simulink model "FO_CTDNN_P_Bia_Para_0_V1"  (R2021b)
settings: Solver=ode5  StartTime=0.0  StopTime=40  FixedStep=0.005  RelTol=1e-3
(part 1 of 2)
settings Model: Creator=a1752760  LastModifiedBy=a1752760
settings SolverCC: AlgebraicLoopSolver=TrustRegion
settings DebuggingCC: SFMachineParentedDataDiag=warning

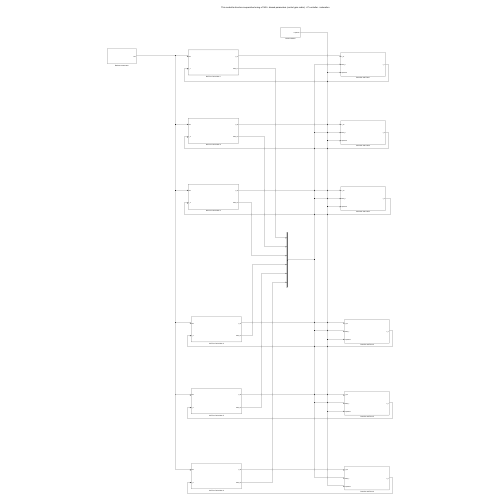
[thumbnail: Simulink's stored preview of the top-level diagram]
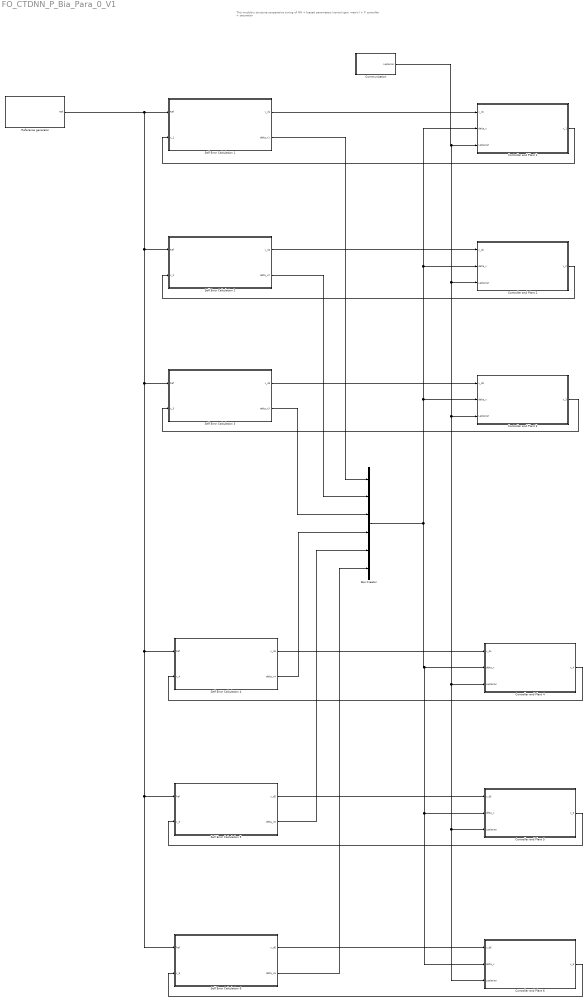
== system FO_CTDNN_P_Bia_Para_0_V1 ==
  note: This module's structure:cooperative tuning of NN + biased parameters (control gain matrix) + P controller + saturation
  Bus Creator : BusCreator  Inputs=6
  Communication : Subsystem
  Controller and Plant 1 : Subsystem  mask{InitialCondition=[-0.2;-0.7;-pi/4], UpperLimit=0.25, LowerLimit=-0.25}
      mask prompts: InitialCondition "Simulink:blkprm_prompts:IntegratorInitCond"; UpperLimit "Simulink:blkprm_prompts:SaturateUpLim"; LowerLimit "Simulink:blkprm_prompts:SaturateLowLim"
      mask TypeOptions InitialCondition: x_int/InitialCondition
      mask TypeOptions UpperLimit: Saturation/UpperLimit
      mask TypeOptions LowerLimit: Saturation/LowerLimit
      mask DialogControl InitialCondition Prompt: Initial condition:
      mask DialogControl UpperLimit Prompt: Upper limit:
      mask DialogControl LowerLimit Prompt: Lower limit:
  Controller and Plant 2 : Subsystem  mask{InitialCondition=[1.6;3.6;-pi/5], UpperLimit=0.25, LowerLimit=-0.25}
      mask prompts: InitialCondition "Simulink:blkprm_prompts:IntegratorInitCond"; UpperLimit "Simulink:blkprm_prompts:SaturateUpLim"; LowerLimit "Simulink:blkprm_prompts:SaturateLowLim"
      mask TypeOptions InitialCondition: x_int/InitialCondition
      mask TypeOptions UpperLimit: Saturation/UpperLimit
      mask TypeOptions LowerLimit: Saturation/LowerLimit
      mask DialogControl InitialCondition Prompt: Initial condition:
      mask DialogControl UpperLimit Prompt: Upper limit:
      mask DialogControl LowerLimit Prompt: Lower limit:
  Controller and Plant 3 : Subsystem  mask{InitialCondition=[-4;-2.4;pi/3], UpperLimit=0.25, LowerLimit=-0.25}
      mask prompts: InitialCondition "Simulink:blkprm_prompts:IntegratorInitCond"; UpperLimit "Simulink:blkprm_prompts:SaturateUpLim"; LowerLimit "Simulink:blkprm_prompts:SaturateLowLim"
      mask TypeOptions InitialCondition: x_int/InitialCondition
      mask TypeOptions UpperLimit: Saturation/UpperLimit
      mask TypeOptions LowerLimit: Saturation/LowerLimit
      mask DialogControl InitialCondition Prompt: Initial condition:
      mask DialogControl UpperLimit Prompt: Upper limit:
      mask DialogControl LowerLimit Prompt: Lower limit:
  Controller and Plant 4 : Subsystem  mask{InitialCondition=[-1.9;-1.1;pi/4], UpperLimit=0.25, LowerLimit=-0.25}
      mask prompts: InitialCondition "Simulink:blkprm_prompts:IntegratorInitCond"; UpperLimit "Simulink:blkprm_prompts:SaturateUpLim"; LowerLimit "Simulink:blkprm_prompts:SaturateLowLim"
      mask TypeOptions InitialCondition: x_int/InitialCondition
      mask TypeOptions UpperLimit: Saturation/UpperLimit
      mask TypeOptions LowerLimit: Saturation/LowerLimit
      mask DialogControl InitialCondition Prompt: Initial condition:
      mask DialogControl UpperLimit Prompt: Upper limit:
      mask DialogControl LowerLimit Prompt: Lower limit:
  Controller and Plant 5 : Subsystem  mask{InitialCondition=[-1.6;-4.6;-pi/3], UpperLimit=0.25, LowerLimit=-0.25}
      mask prompts: InitialCondition "Simulink:blkprm_prompts:IntegratorInitCond"; UpperLimit "Simulink:blkprm_prompts:SaturateUpLim"; LowerLimit "Simulink:blkprm_prompts:SaturateLowLim"
      mask TypeOptions InitialCondition: x_int/InitialCondition
      mask TypeOptions UpperLimit: Saturation/UpperLimit
      mask TypeOptions LowerLimit: Saturation/LowerLimit
      mask DialogControl InitialCondition Prompt: Initial condition:
      mask DialogControl UpperLimit Prompt: Upper limit:
      mask DialogControl LowerLimit Prompt: Lower limit:
  Controller and Plant 6 : Subsystem  mask{InitialCondition=[3.6;-1.5;-pi/6], UpperLimit=0.25, LowerLimit=-0.25}
      mask prompts: InitialCondition "Simulink:blkprm_prompts:IntegratorInitCond"; UpperLimit "Simulink:blkprm_prompts:SaturateUpLim"; LowerLimit "Simulink:blkprm_prompts:SaturateLowLim"
      mask TypeOptions InitialCondition: x_int/InitialCondition
      mask TypeOptions UpperLimit: Saturation/UpperLimit
      mask TypeOptions LowerLimit: Saturation/LowerLimit
      mask DialogControl InitialCondition Prompt: Initial condition:
      mask DialogControl UpperLimit Prompt: Upper limit:
      mask DialogControl LowerLimit Prompt: Lower limit:
  Reference generator : Subsystem
  Self Error Calculation 1 : Subsystem
  Self Error Calculation 2 : Subsystem
  Self Error Calculation 3 : Subsystem
  Self Error Calculation 4 : Subsystem
  Self Error Calculation 5 : Subsystem
  Self Error Calculation 6 : Subsystem
  wires:
  Reference generator/1(Ref) -> Self Error Calculation 6/1(Ref), Self Error Calculation 5/1(Ref), Self Error Calculation 4/1(Ref), Self Error Calculation 3/1(Ref), Self Error Calculation 2/1(Ref), Self Error Calculation 1/1(Ref)
  Self Error Calculation 1/1(v_d1) -> Controller and Plant 1/1(v_d1)
  Controller and Plant 1/1(x_1) -> Self Error Calculation 1/2(x_1)
  Controller and Plant 2/1(x_2) -> Self Error Calculation 2/2(x_2)
  Self Error Calculation 2/1(v_d2) -> Controller and Plant 2/1(v_d2)
  Controller and Plant 3/1(x_3) -> Self Error Calculation 3/2(x_3)
  Self Error Calculation 3/1(v_d3) -> Controller and Plant 3/1(v_d3)
  Controller and Plant 4/1(x_4) -> Self Error Calculation 4/2(x_4)
  Self Error Calculation 4/1(v_d4) -> Controller and Plant 4/1(v_d4)
  Controller and Plant 5/1(x_5) -> Self Error Calculation 5/2(x_5)
  Self Error Calculation 5/1(v_d5) -> Controller and Plant 5/1(v_d5)
  Controller and Plant 6/1(x_6) -> Self Error Calculation 6/2(x_6)
  Self Error Calculation 6/1(v_d6) -> Controller and Plant 6/1(v_d6)
  Self Error Calculation 1/2(delta_x1) -> Bus Creator/1
  Self Error Calculation 2/2(delta_x2) -> Bus Creator/2
  Self Error Calculation 3/2(delta_x3) -> Bus Creator/3
  Self Error Calculation 4/2(delta_x4) -> Bus Creator/4
  Self Error Calculation 5/2(delta_x5) -> Bus Creator/5
  Self Error Calculation 6/2(delta_x6) -> Bus Creator/6
  Bus Creator/1 -> Controller and Plant 4/2(delta_x), Controller and Plant 6/2(delta_x), Controller and Plant 5/2(delta_x), Controller and Plant 3/2(delta_x), Controller and Plant 2/2(delta_x), Controller and Plant 1/2(delta_x)
  Communication/1(Laplacian) -> Controller and Plant 6/3(Laplacian), Controller and Plant 5/3(Laplacian), Controller and Plant 4/3(Laplacian), Controller and Plant 3/3(Laplacian), Controller and Plant 2/3(Laplacian), Controller and Plant 1/3(Laplacian)

== system FO_CTDNN_P_Bia_Para_0_V1/Communication ==
  Add : Sum
  Communication Topology : Constant  Value=[2,0,-1,-1,0,0;-1,1,0,0,0,0;0,-1,2,-1,0,0;-1,0,0,3,-1,-1;0,0,0,-1,1,0;-1,0,0,0,0,1]  VectorParams1D=off
  Constant : Constant  Value=2  VectorParams1D=off
  Product : Product
  Reference Feeding : Constant  Value=[1,0,0,0,0,0;0,1,0,0,0,0;0,0,1,0,0,0;0,0,0,1,0,0;0,0,0,0,1,0;0,0,0,0,0,1]  VectorParams1D=off
  Laplacian : Outport  VectorParamsAs1DForOutWhenUnconnected=off
  wires:
  Constant/1 -> Product/2
  Reference Feeding/1 -> Product/1
  Communication Topology/1 -> Add/1
  Product/1 -> Add/2
  Add/1 -> Laplacian/1

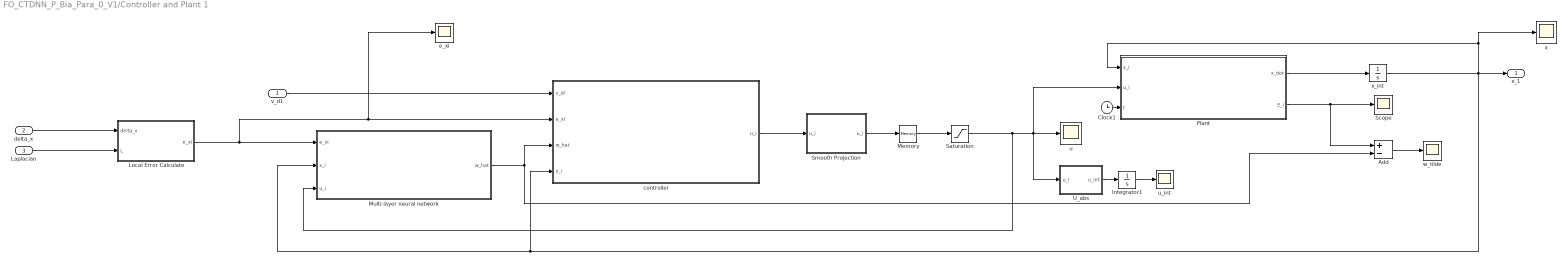
== system FO_CTDNN_P_Bia_Para_0_V1/Controller and Plant 1 ==
  v_d1 : Inport
  delta_x : Inport  Port=2
  Laplacian : Inport  Port=3
  Add : Sum  Inputs=+-
  Clock1 : Clock
  Integrator1 : Integrator
  Local Error Calculate : MATLAB Function  TreatAsAtomicUnit=on
  Memory : Memory  InitialCondition=[0;0;0]
  Multi-layer neural network : Subsystem
  Plant : MATLAB Function  TreatAsAtomicUnit=on
  Saturation : Saturate  UpperLimit=UpperLimit  LowerLimit=LowerLimit
  Scope : Scope
  Smooth Projection : MATLAB Function  TreatAsAtomicUnit=on
  U_abs : MATLAB Function  TreatAsAtomicUnit=on
  controller : MATLAB Function  TreatAsAtomicUnit=on
  e_xi : Scope
  u : Scope
  u_int : Scope
  w_tilde : Scope
  x : Scope
  x_int : Integrator  InitialCondition=InitialCondition
  x_1 : Outport
  wires:
  Add/1 -> w_tilde/1
  Plant/2(E_i) -> Scope/1, Add/1
  Multi-layer neural network/1(w_hat) -> controller/3(w_hat), Add/2
  Clock1/1 -> Plant/3(t)
  Plant/1(x_dot) -> x_int/1
  Memory/1 -> Saturation/1
  x_int/1 -> x_1/1, x/1, Plant/1(x_i), controller/4(x_i), Multi-layer neural network/2(x_i)
  v_d1/1 -> controller/1(v_di)
  controller/1(u_i) -> Smooth Projection/1("u_i ")
  Smooth Projection/1(u_i) -> Memory/1
  Local Error Calculate/1(e_xi) -> e_xi/1, controller/2(e_xi), Multi-layer neural network/1(e_xi)
  delta_x/1 -> Local Error Calculate/1(delta_x)
  Laplacian/1 -> Local Error Calculate/2(L)
  Integrator1/1 -> u_int/1
  Saturation/1 -> Multi-layer neural network/3(u_i), U_abs/1(u_i), Plant/2(u_i), u/1
  U_abs/1(u_int) -> Integrator1/1

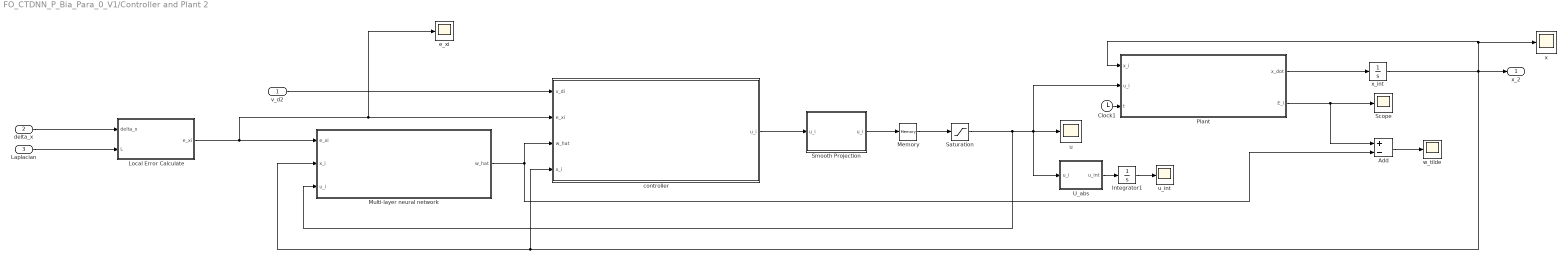
== system FO_CTDNN_P_Bia_Para_0_V1/Controller and Plant 2 ==
  v_d2 : Inport
  delta_x : Inport  Port=2
  Laplacian : Inport  Port=3
  Add : Sum  Inputs=+-
  Clock1 : Clock
  Integrator1 : Integrator
  Local Error Calculate : MATLAB Function  TreatAsAtomicUnit=on
  Memory : Memory  InitialCondition=[0;0;0]
  Multi-layer neural network : Subsystem
  Plant : MATLAB Function  TreatAsAtomicUnit=on
  Saturation : Saturate  UpperLimit=UpperLimit  LowerLimit=LowerLimit
  Scope : Scope
  Smooth Projection : MATLAB Function  TreatAsAtomicUnit=on
  U_abs : MATLAB Function  TreatAsAtomicUnit=on
  controller : MATLAB Function  TreatAsAtomicUnit=on
  e_xi : Scope
  u : Scope
  u_int : Scope
  w_tilde : Scope
  x : Scope
  x_int : Integrator  InitialCondition=InitialCondition
  x_2 : Outport
  wires:
  Add/1 -> w_tilde/1
  Plant/2(E_i) -> Scope/1, Add/1
  Multi-layer neural network/1(w_hat) -> controller/3(w_hat), Add/2
  Clock1/1 -> Plant/3(t)
  Plant/1(x_dot) -> x_int/1
  Memory/1 -> Saturation/1
  x_int/1 -> x_2/1, Plant/1(x_i), x/1, controller/4(x_i), Multi-layer neural network/2(x_i)
  v_d2/1 -> controller/1(v_di)
  controller/1(u_i) -> Smooth Projection/1("u_i ")
  Smooth Projection/1(u_i) -> Memory/1
  Local Error Calculate/1(e_xi) -> e_xi/1, controller/2(e_xi), Multi-layer neural network/1(e_xi)
  delta_x/1 -> Local Error Calculate/1(delta_x)
  Laplacian/1 -> Local Error Calculate/2(L)
  Integrator1/1 -> u_int/1
  Saturation/1 -> Multi-layer neural network/3(u_i), U_abs/1(u_i), Plant/2(u_i), u/1
  U_abs/1(u_int) -> Integrator1/1

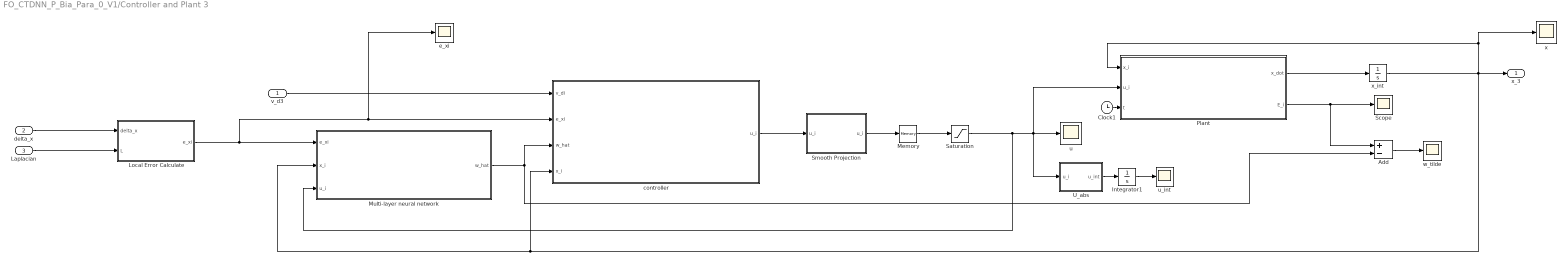
== system FO_CTDNN_P_Bia_Para_0_V1/Controller and Plant 3 ==
  v_d3 : Inport
  delta_x : Inport  Port=2
  Laplacian : Inport  Port=3
  Add : Sum  Inputs=+-
  Clock1 : Clock
  Integrator1 : Integrator
  Local Error Calculate : MATLAB Function  TreatAsAtomicUnit=on
  Memory : Memory  InitialCondition=[0;0;0]
  Multi-layer neural network : Subsystem
  Plant : MATLAB Function  TreatAsAtomicUnit=on
  Saturation : Saturate  UpperLimit=UpperLimit  LowerLimit=LowerLimit
  Scope : Scope
  Smooth Projection : MATLAB Function  TreatAsAtomicUnit=on
  U_abs : MATLAB Function  TreatAsAtomicUnit=on
  controller : MATLAB Function  TreatAsAtomicUnit=on
  e_xi : Scope
  u : Scope
  u_int : Scope
  w_tilde : Scope
  x : Scope
  x_int : Integrator  InitialCondition=InitialCondition
  x_3 : Outport
  wires:
  Add/1 -> w_tilde/1
  Plant/2(E_i) -> Scope/1, Add/1
  Multi-layer neural network/1(w_hat) -> controller/3(w_hat), Add/2
  Clock1/1 -> Plant/3(t)
  Plant/1(x_dot) -> x_int/1
  Memory/1 -> Saturation/1
  x_int/1 -> x_3/1, x/1, Plant/1(x_i), controller/4(x_i), Multi-layer neural network/2(x_i)
  v_d3/1 -> controller/1(v_di)
  controller/1(u_i) -> Smooth Projection/1("u_i ")
  Smooth Projection/1(u_i) -> Memory/1
  Local Error Calculate/1(e_xi) -> e_xi/1, controller/2(e_xi), Multi-layer neural network/1(e_xi)
  delta_x/1 -> Local Error Calculate/1(delta_x)
  Laplacian/1 -> Local Error Calculate/2(L)
  Integrator1/1 -> u_int/1
  Saturation/1 -> Multi-layer neural network/3(u_i), U_abs/1(u_i), Plant/2(u_i), u/1
  U_abs/1(u_int) -> Integrator1/1

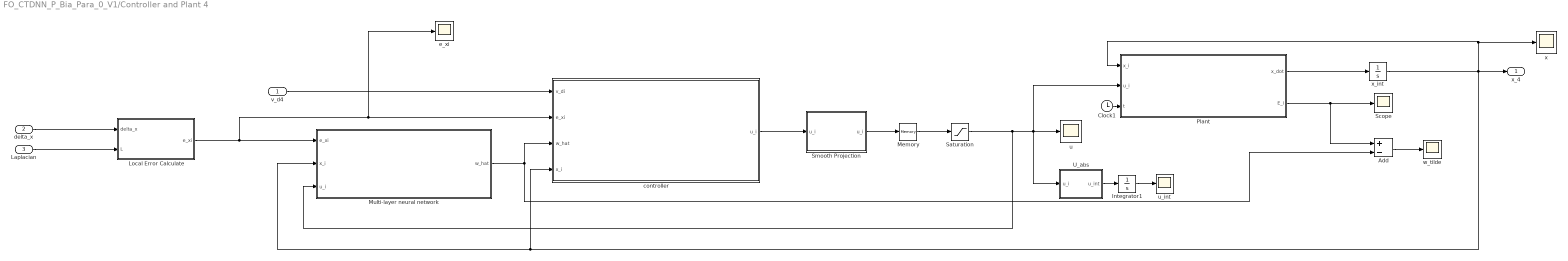
== system FO_CTDNN_P_Bia_Para_0_V1/Controller and Plant 4 ==
  v_d4 : Inport
  delta_x : Inport  Port=2
  Laplacian : Inport  Port=3
  Add : Sum  Inputs=+-
  Clock1 : Clock
  Integrator1 : Integrator
  Local Error Calculate : MATLAB Function  TreatAsAtomicUnit=on
  Memory : Memory  InitialCondition=[0;0;0]
  Multi-layer neural network : Subsystem
  Plant : MATLAB Function  TreatAsAtomicUnit=on
  Saturation : Saturate  UpperLimit=UpperLimit  LowerLimit=LowerLimit
  Scope : Scope
  Smooth Projection : MATLAB Function  TreatAsAtomicUnit=on
  U_abs : MATLAB Function  TreatAsAtomicUnit=on
  controller : MATLAB Function  TreatAsAtomicUnit=on
  e_xi : Scope
  u : Scope
  u_int : Scope
  w_tilde : Scope
  x : Scope
  x_int : Integrator  InitialCondition=InitialCondition
  x_4 : Outport
  wires:
  Add/1 -> w_tilde/1
  Plant/2(E_i) -> Scope/1, Add/1
  Multi-layer neural network/1(w_hat) -> controller/3(w_hat), Add/2
  Clock1/1 -> Plant/3(t)
  Plant/1(x_dot) -> x_int/1
  Memory/1 -> Saturation/1
  x_int/1 -> x_4/1, Plant/1(x_i), x/1, controller/4(x_i), Multi-layer neural network/2(x_i)
  v_d4/1 -> controller/1(v_di)
  controller/1(u_i) -> Smooth Projection/1("u_i ")
  Smooth Projection/1(u_i) -> Memory/1
  Local Error Calculate/1(e_xi) -> e_xi/1, controller/2(e_xi), Multi-layer neural network/1(e_xi)
  delta_x/1 -> Local Error Calculate/1(delta_x)
  Laplacian/1 -> Local Error Calculate/2(L)
  Integrator1/1 -> u_int/1
  Saturation/1 -> Multi-layer neural network/3(u_i), U_abs/1(u_i), Plant/2(u_i), u/1
  U_abs/1(u_int) -> Integrator1/1

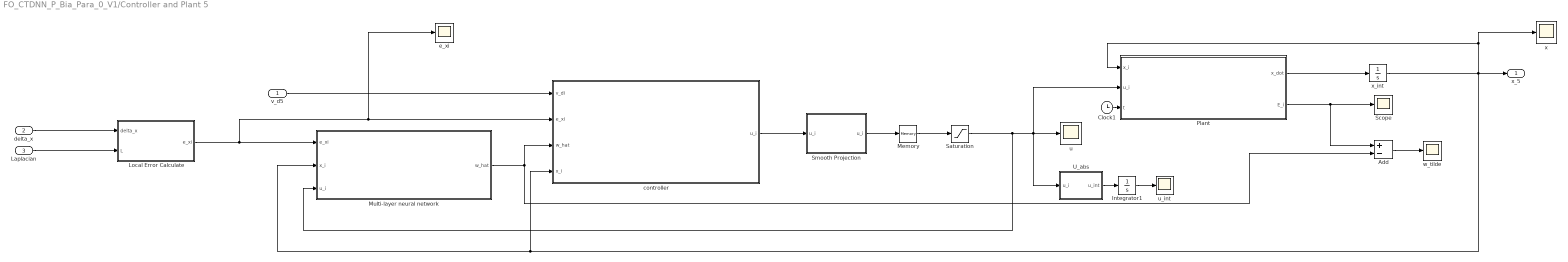
== system FO_CTDNN_P_Bia_Para_0_V1/Controller and Plant 5 ==
  v_d5 : Inport
  delta_x : Inport  Port=2
  Laplacian : Inport  Port=3
  Add : Sum  Inputs=+-
  Clock1 : Clock
  Integrator1 : Integrator
  Local Error Calculate : MATLAB Function  TreatAsAtomicUnit=on
  Memory : Memory  InitialCondition=[0;0;0]
  Multi-layer neural network : Subsystem
  Plant : MATLAB Function  TreatAsAtomicUnit=on
  Saturation : Saturate  UpperLimit=UpperLimit  LowerLimit=LowerLimit
  Scope : Scope
  Smooth Projection : MATLAB Function  TreatAsAtomicUnit=on
  U_abs : MATLAB Function  TreatAsAtomicUnit=on
  controller : MATLAB Function  TreatAsAtomicUnit=on
  e_xi : Scope
  u : Scope
  u_int : Scope
  w_tilde : Scope
  x : Scope
  x_int : Integrator  InitialCondition=InitialCondition
  x_5 : Outport
  wires:
  Add/1 -> w_tilde/1
  Plant/2(E_i) -> Scope/1, Add/1
  Multi-layer neural network/1(w_hat) -> controller/3(w_hat), Add/2
  Clock1/1 -> Plant/3(t)
  Plant/1(x_dot) -> x_int/1
  Memory/1 -> Saturation/1
  x_int/1 -> x_5/1, x/1, Plant/1(x_i), controller/4(x_i), Multi-layer neural network/2(x_i)
  v_d5/1 -> controller/1(v_di)
  controller/1(u_i) -> Smooth Projection/1("u_i ")
  Smooth Projection/1(u_i) -> Memory/1
  Local Error Calculate/1(e_xi) -> e_xi/1, controller/2(e_xi), Multi-layer neural network/1(e_xi)
  delta_x/1 -> Local Error Calculate/1(delta_x)
  Laplacian/1 -> Local Error Calculate/2(L)
  Integrator1/1 -> u_int/1
  Saturation/1 -> Multi-layer neural network/3(u_i), U_abs/1(u_i), Plant/2(u_i), u/1
  U_abs/1(u_int) -> Integrator1/1

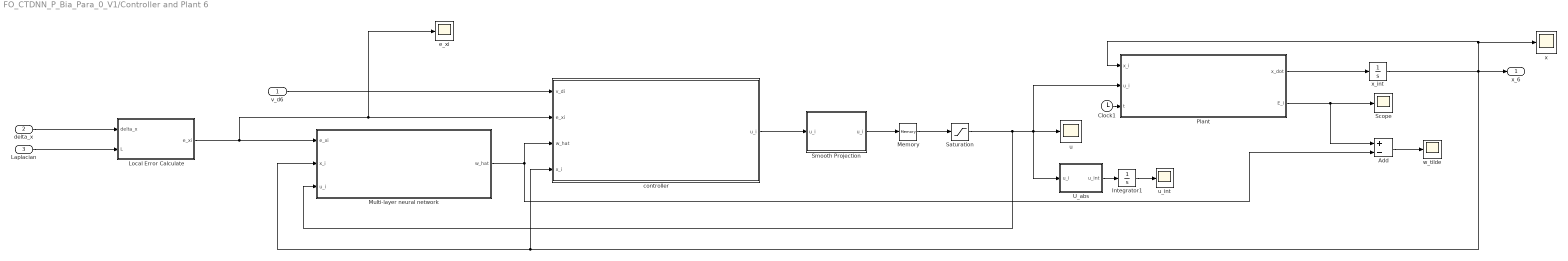
== system FO_CTDNN_P_Bia_Para_0_V1/Controller and Plant 6 ==
  v_d6 : Inport
  delta_x : Inport  Port=2
  Laplacian : Inport  Port=3
  Add : Sum  Inputs=+-
  Clock1 : Clock
  Integrator1 : Integrator
  Local Error Calculate : MATLAB Function  TreatAsAtomicUnit=on
  Memory : Memory  InitialCondition=[0;0;0]
  Multi-layer neural network : Subsystem
  Plant : MATLAB Function  TreatAsAtomicUnit=on
  Saturation : Saturate  UpperLimit=UpperLimit  LowerLimit=LowerLimit
  Scope : Scope
  Smooth Projection : MATLAB Function  TreatAsAtomicUnit=on
  U_abs : MATLAB Function  TreatAsAtomicUnit=on
  controller : MATLAB Function  TreatAsAtomicUnit=on
  e_xi : Scope
  u : Scope
  u_int : Scope
  w_tilde : Scope
  x : Scope
  x_int : Integrator  InitialCondition=InitialCondition
  x_6 : Outport
  wires:
  Add/1 -> w_tilde/1
  Plant/2(E_i) -> Scope/1, Add/1
  Multi-layer neural network/1(w_hat) -> controller/3(w_hat), Add/2
  Clock1/1 -> Plant/3(t)
  Plant/1(x_dot) -> x_int/1
  Memory/1 -> Saturation/1
  x_int/1 -> x_6/1, Plant/1(x_i), x/1, controller/4(x_i), Multi-layer neural network/2(x_i)
  v_d6/1 -> controller/1(v_di)
  controller/1(u_i) -> Smooth Projection/1("u_i ")
  Smooth Projection/1(u_i) -> Memory/1
  Local Error Calculate/1(e_xi) -> e_xi/1, controller/2(e_xi), Multi-layer neural network/1(e_xi)
  delta_x/1 -> Local Error Calculate/1(delta_x)
  Laplacian/1 -> Local Error Calculate/2(L)
  Integrator1/1 -> u_int/1
  Saturation/1 -> Multi-layer neural network/3(u_i), U_abs/1(u_i), Plant/2(u_i), u/1
  U_abs/1(u_int) -> Integrator1/1

== system FO_CTDNN_P_Bia_Para_0_V1/Reference generator ==
  Bus Creator : BusCreator  Inputs=2
  Clock : Clock
  reference : MATLAB Function  TreatAsAtomicUnit=on
  reference1 : MATLAB Function  TreatAsAtomicUnit=on
  Ref : Outport
  wires:
  Clock/1 -> reference1/1(t), reference/1(t)
  reference/1(xd) -> Bus Creator/1
  reference1/1(vd) -> Bus Creator/2
  Bus Creator/1 -> Ref/1

== system FO_CTDNN_P_Bia_Para_0_V1/Self Error Calculation 1 ==
  Ref : Inport
  x_1 : Inport  Port=2
  Scope : Scope
  error_calculation : MATLAB Function  TreatAsAtomicUnit=on
  v_d1 : Outport
  delta_x1 : Outport  Port=2
  wires:
  Ref/1 -> error_calculation/1(ref)
  x_1/1 -> error_calculation/2(x_i)
  error_calculation/1(v_di) -> v_d1/1
  error_calculation/2(delta_x1) -> Scope/1, delta_x1/1

== system FO_CTDNN_P_Bia_Para_0_V1/Self Error Calculation 2 ==
  Ref : Inport
  x_2 : Inport  Port=2
  Scope : Scope
  error_calculation : MATLAB Function  TreatAsAtomicUnit=on
  v_d2 : Outport
  delta_x2 : Outport  Port=2
  wires:
  Ref/1 -> error_calculation/1(ref)
  x_2/1 -> error_calculation/2(x_i)
  error_calculation/1(v_di) -> v_d2/1
  error_calculation/2(delta_x2) -> Scope/1, delta_x2/1

== system FO_CTDNN_P_Bia_Para_0_V1/Self Error Calculation 3 ==
  Ref : Inport
  x_3 : Inport  Port=2
  Scope : Scope
  error_calculation : MATLAB Function  TreatAsAtomicUnit=on
  v_d3 : Outport
  delta_x3 : Outport  Port=2
  wires:
  Ref/1 -> error_calculation/1(ref)
  x_3/1 -> error_calculation/2(x_i)
  error_calculation/1(v_di) -> v_d3/1
  error_calculation/2(delta_x3) -> Scope/1, delta_x3/1

== system FO_CTDNN_P_Bia_Para_0_V1/Self Error Calculation 4 ==
  Ref : Inport
  x_4 : Inport  Port=2
  Scope : Scope
  error_calculation : MATLAB Function  TreatAsAtomicUnit=on
  v_d4 : Outport
  delta_x4 : Outport  Port=2
  wires:
  Ref/1 -> error_calculation/1(ref)
  x_4/1 -> error_calculation/2(x_i)
  error_calculation/1(v_di) -> v_d4/1
  error_calculation/2(delta_x4) -> Scope/1, delta_x4/1

== system FO_CTDNN_P_Bia_Para_0_V1/Self Error Calculation 5 ==
  Ref : Inport
  x_5 : Inport  Port=2
  Scope : Scope
  error_calculation : MATLAB Function  TreatAsAtomicUnit=on
  v_d5 : Outport
  delta_x5 : Outport  Port=2
  wires:
  Ref/1 -> error_calculation/1(ref)
  x_5/1 -> error_calculation/2(x_i)
  error_calculation/1(v_di) -> v_d5/1
  error_calculation/2(delta_x5) -> Scope/1, delta_x5/1

== system FO_CTDNN_P_Bia_Para_0_V1/Self Error Calculation 6 ==
  Ref : Inport
  x_6 : Inport  Port=2
  Scope : Scope
  error_calculation : MATLAB Function  TreatAsAtomicUnit=on
  v_d6 : Outport
  delta_x6 : Outport  Port=2
  wires:
  Ref/1 -> error_calculation/1(ref)
  x_6/1 -> error_calculation/2(x_i)
  error_calculation/1(v_di) -> v_d6/1
  error_calculation/2(delta_x6) -> Scope/1, delta_x6/1

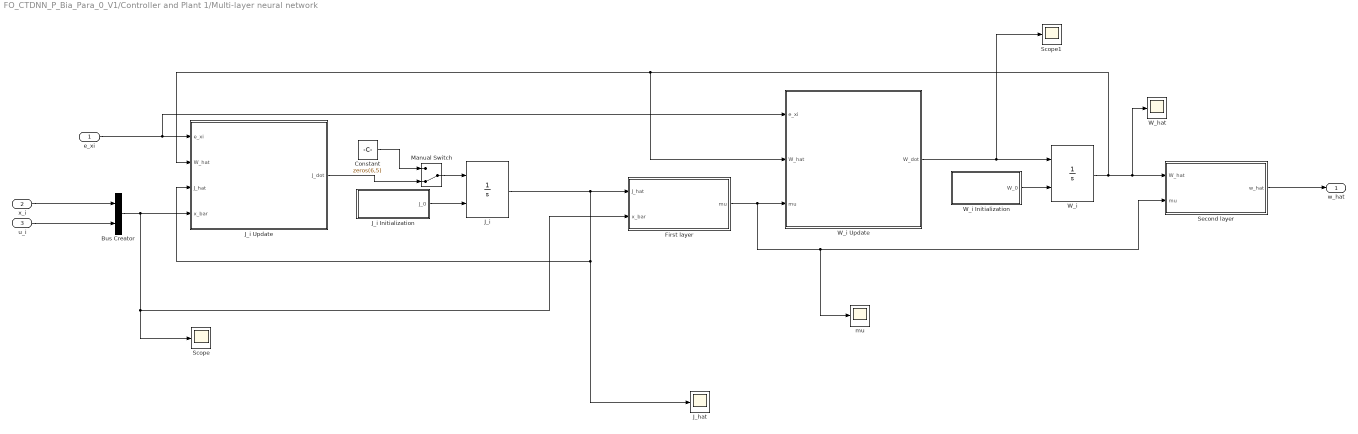
== system FO_CTDNN_P_Bia_Para_0_V1/Controller and Plant 1/Multi-layer neural network ==
  e_xi : Inport
  x_i : Inport  Port=2  PortDimensions=[3,1]
  u_i : Inport  Port=3  PortDimensions=[3,1]
  Bus Creator : BusCreator  Inputs=2
  Constant : Constant  Value=zeros(6,5)
  First layer : MATLAB Function  TreatAsAtomicUnit=on
  J_hat : Scope
  J_i : Integrator  InitialConditionSource=external
  J_i Initialization : MATLAB Function  TreatAsAtomicUnit=on
  J_i Update : MATLAB Function  TreatAsAtomicUnit=on
  Manual Switch : ManualSwitch  CurrentSetting=0
  Scope : Scope
  Scope1 : Scope
  Second layer : MATLAB Function  TreatAsAtomicUnit=on
  W_hat : Scope
  W_i : Integrator  InitialConditionSource=external
  W_i Initialization : MATLAB Function  TreatAsAtomicUnit=on
  W_i Update : MATLAB Function  TreatAsAtomicUnit=on
  mu : Scope
  w_hat : Outport
  wires:
  e_xi/1 -> W_i Update/1(e_xi), J_i Update/1(e_xi)
  W_i/1 -> W_hat/1, Second layer/1(W_hat), W_i Update/2(W_hat), J_i Update/2(W_hat)
  W_i Update/1(W_dot) -> Scope1/1, W_i/1
  W_i Initialization/1(W_0) -> W_i/2
  J_i Initialization/1(J_0) -> J_i/2
  First layer/1(mu) -> mu/1, Second layer/2(mu), W_i Update/3(mu)
  Second layer/1(w_hat) -> w_hat/1
  J_i/1 -> J_i Update/3(J_hat), J_hat/1, First layer/1(J_hat)
  Bus Creator/1 -> Scope/1, First layer/2(x_bar), J_i Update/4(x_bar)
  x_i/1 -> Bus Creator/1
  u_i/1 -> Bus Creator/2
  J_i Update/1(J_dot) -> Manual Switch/2
  Constant/1 -> Manual Switch/1
  Manual Switch/1 -> J_i/1

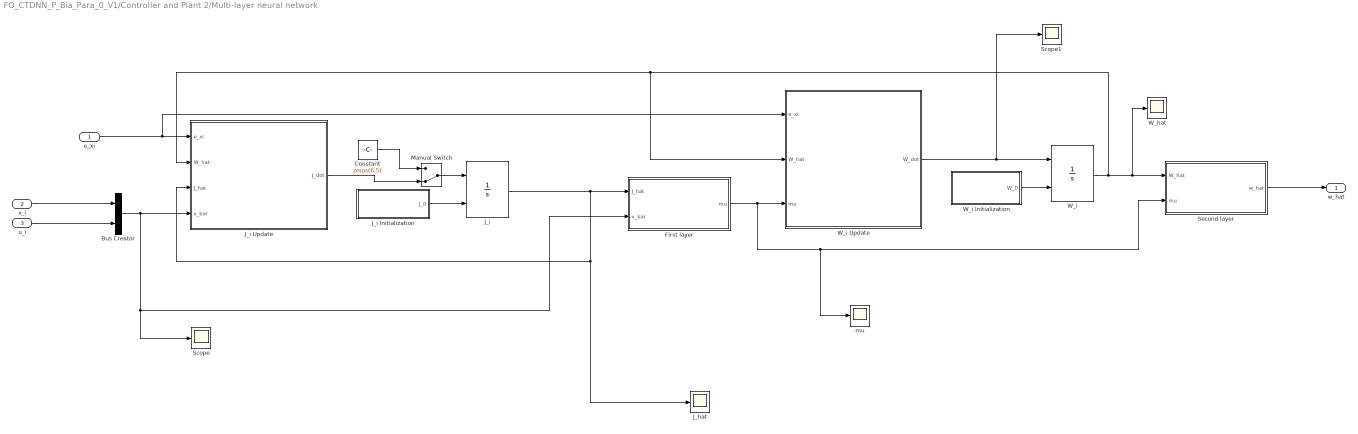
== system FO_CTDNN_P_Bia_Para_0_V1/Controller and Plant 2/Multi-layer neural network ==
  e_xi : Inport
  x_i : Inport  Port=2  PortDimensions=[3,1]
  u_i : Inport  Port=3  PortDimensions=[3,1]
  Bus Creator : BusCreator  Inputs=2
  Constant : Constant  Value=zeros(6,5)
  First layer : MATLAB Function  TreatAsAtomicUnit=on
  J_hat : Scope
  J_i : Integrator  InitialConditionSource=external
  J_i Initialization : MATLAB Function  TreatAsAtomicUnit=on
  J_i Update : MATLAB Function  TreatAsAtomicUnit=on
  Manual Switch : ManualSwitch  CurrentSetting=0
  Scope : Scope
  Scope1 : Scope
  Second layer : MATLAB Function  TreatAsAtomicUnit=on
  W_hat : Scope
  W_i : Integrator  InitialConditionSource=external
  W_i Initialization : MATLAB Function  TreatAsAtomicUnit=on
  W_i Update : MATLAB Function  TreatAsAtomicUnit=on
  mu : Scope
  w_hat : Outport
  wires:
  e_xi/1 -> W_i Update/1(e_xi), J_i Update/1(e_xi)
  W_i/1 -> W_hat/1, Second layer/1(W_hat), W_i Update/2(W_hat), J_i Update/2(W_hat)
  W_i Update/1(W_dot) -> Scope1/1, W_i/1
  W_i Initialization/1(W_0) -> W_i/2
  J_i Initialization/1(J_0) -> J_i/2
  First layer/1(mu) -> mu/1, Second layer/2(mu), W_i Update/3(mu)
  Second layer/1(w_hat) -> w_hat/1
  J_i/1 -> J_i Update/3(J_hat), J_hat/1, First layer/1(J_hat)
  Bus Creator/1 -> Scope/1, First layer/2(x_bar), J_i Update/4(x_bar)
  x_i/1 -> Bus Creator/1
  u_i/1 -> Bus Creator/2
  J_i Update/1(J_dot) -> Manual Switch/2
  Constant/1 -> Manual Switch/1
  Manual Switch/1 -> J_i/1

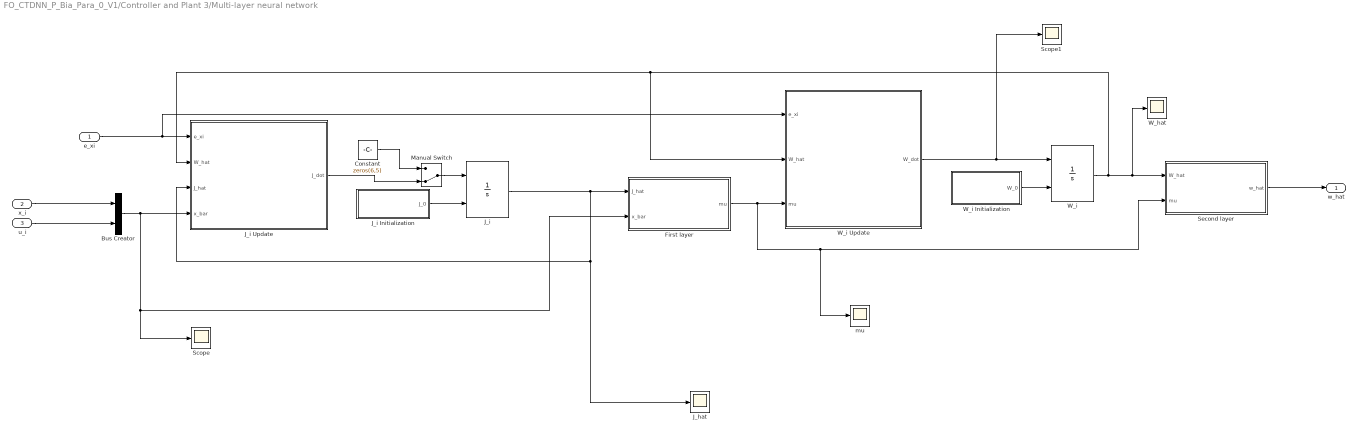
== system FO_CTDNN_P_Bia_Para_0_V1/Controller and Plant 3/Multi-layer neural network ==
  e_xi : Inport
  x_i : Inport  Port=2  PortDimensions=[3,1]
  u_i : Inport  Port=3  PortDimensions=[3,1]
  Bus Creator : BusCreator  Inputs=2
  Constant : Constant  Value=zeros(6,5)
  First layer : MATLAB Function  TreatAsAtomicUnit=on
  J_hat : Scope
  J_i : Integrator  InitialConditionSource=external
  J_i Initialization : MATLAB Function  TreatAsAtomicUnit=on
  J_i Update : MATLAB Function  TreatAsAtomicUnit=on
  Manual Switch : ManualSwitch  CurrentSetting=0
  Scope : Scope
  Scope1 : Scope
  Second layer : MATLAB Function  TreatAsAtomicUnit=on
  W_hat : Scope
  W_i : Integrator  InitialConditionSource=external
  W_i Initialization : MATLAB Function  TreatAsAtomicUnit=on
  W_i Update : MATLAB Function  TreatAsAtomicUnit=on
  mu : Scope
  w_hat : Outport
  wires:
  e_xi/1 -> W_i Update/1(e_xi), J_i Update/1(e_xi)
  W_i/1 -> W_hat/1, Second layer/1(W_hat), W_i Update/2(W_hat), J_i Update/2(W_hat)
  W_i Update/1(W_dot) -> Scope1/1, W_i/1
  W_i Initialization/1(W_0) -> W_i/2
  J_i Initialization/1(J_0) -> J_i/2
  First layer/1(mu) -> mu/1, Second layer/2(mu), W_i Update/3(mu)
  Second layer/1(w_hat) -> w_hat/1
  J_i/1 -> J_i Update/3(J_hat), J_hat/1, First layer/1(J_hat)
  Bus Creator/1 -> Scope/1, First layer/2(x_bar), J_i Update/4(x_bar)
  x_i/1 -> Bus Creator/1
  u_i/1 -> Bus Creator/2
  J_i Update/1(J_dot) -> Manual Switch/2
  Constant/1 -> Manual Switch/1
  Manual Switch/1 -> J_i/1

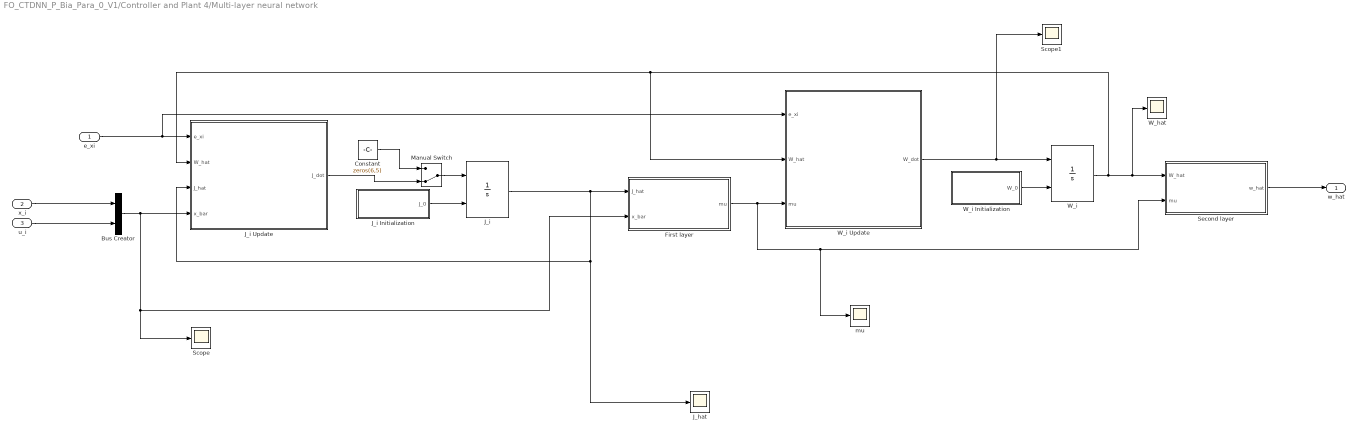
== system FO_CTDNN_P_Bia_Para_0_V1/Controller and Plant 4/Multi-layer neural network ==
  e_xi : Inport
  x_i : Inport  Port=2  PortDimensions=[3,1]
  u_i : Inport  Port=3  PortDimensions=[3,1]
  Bus Creator : BusCreator  Inputs=2
  Constant : Constant  Value=zeros(6,5)
  First layer : MATLAB Function  TreatAsAtomicUnit=on
  J_hat : Scope
  J_i : Integrator  InitialConditionSource=external
  J_i Initialization : MATLAB Function  TreatAsAtomicUnit=on
  J_i Update : MATLAB Function  TreatAsAtomicUnit=on
  Manual Switch : ManualSwitch  CurrentSetting=0
  Scope : Scope
  Scope1 : Scope
  Second layer : MATLAB Function  TreatAsAtomicUnit=on
  W_hat : Scope
  W_i : Integrator  InitialConditionSource=external
  W_i Initialization : MATLAB Function  TreatAsAtomicUnit=on
  W_i Update : MATLAB Function  TreatAsAtomicUnit=on
  mu : Scope
  w_hat : Outport
  wires:
  e_xi/1 -> W_i Update/1(e_xi), J_i Update/1(e_xi)
  W_i/1 -> W_hat/1, Second layer/1(W_hat), W_i Update/2(W_hat), J_i Update/2(W_hat)
  W_i Update/1(W_dot) -> Scope1/1, W_i/1
  W_i Initialization/1(W_0) -> W_i/2
  J_i Initialization/1(J_0) -> J_i/2
  First layer/1(mu) -> mu/1, Second layer/2(mu), W_i Update/3(mu)
  Second layer/1(w_hat) -> w_hat/1
  J_i/1 -> J_i Update/3(J_hat), J_hat/1, First layer/1(J_hat)
  Bus Creator/1 -> Scope/1, First layer/2(x_bar), J_i Update/4(x_bar)
  x_i/1 -> Bus Creator/1
  u_i/1 -> Bus Creator/2
  J_i Update/1(J_dot) -> Manual Switch/2
  Constant/1 -> Manual Switch/1
  Manual Switch/1 -> J_i/1

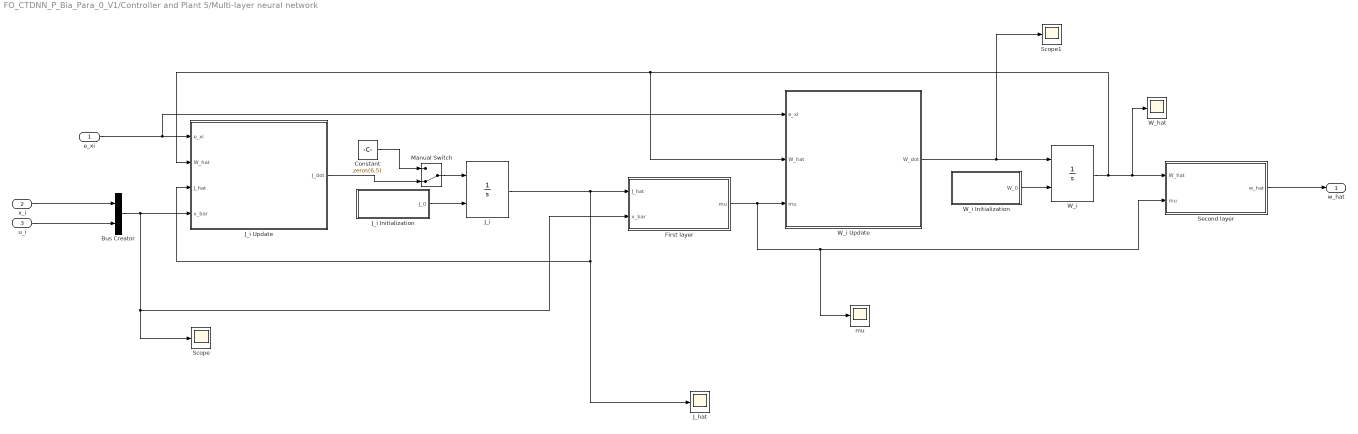
== system FO_CTDNN_P_Bia_Para_0_V1/Controller and Plant 5/Multi-layer neural network ==
  e_xi : Inport
  x_i : Inport  Port=2  PortDimensions=[3,1]
  u_i : Inport  Port=3  PortDimensions=[3,1]
  Bus Creator : BusCreator  Inputs=2
  Constant : Constant  Value=zeros(6,5)
  First layer : MATLAB Function  TreatAsAtomicUnit=on
  J_hat : Scope
  J_i : Integrator  InitialConditionSource=external
  J_i Initialization : MATLAB Function  TreatAsAtomicUnit=on
  J_i Update : MATLAB Function  TreatAsAtomicUnit=on
  Manual Switch : ManualSwitch  CurrentSetting=0
  Scope : Scope
  Scope1 : Scope
  Second layer : MATLAB Function  TreatAsAtomicUnit=on
  W_hat : Scope
  W_i : Integrator  InitialConditionSource=external
  W_i Initialization : MATLAB Function  TreatAsAtomicUnit=on
  W_i Update : MATLAB Function  TreatAsAtomicUnit=on
  mu : Scope
  w_hat : Outport
  wires:
  e_xi/1 -> W_i Update/1(e_xi), J_i Update/1(e_xi)
  W_i/1 -> W_hat/1, Second layer/1(W_hat), W_i Update/2(W_hat), J_i Update/2(W_hat)
  W_i Update/1(W_dot) -> Scope1/1, W_i/1
  W_i Initialization/1(W_0) -> W_i/2
  J_i Initialization/1(J_0) -> J_i/2
  First layer/1(mu) -> mu/1, Second layer/2(mu), W_i Update/3(mu)
  Second layer/1(w_hat) -> w_hat/1
  J_i/1 -> J_i Update/3(J_hat), J_hat/1, First layer/1(J_hat)
  Bus Creator/1 -> Scope/1, First layer/2(x_bar), J_i Update/4(x_bar)
  x_i/1 -> Bus Creator/1
  u_i/1 -> Bus Creator/2
  J_i Update/1(J_dot) -> Manual Switch/2
  Constant/1 -> Manual Switch/1
  Manual Switch/1 -> J_i/1

== system FO_CTDNN_P_Bia_Para_0_V1/Controller and Plant 6/Multi-layer neural network ==
  e_xi : Inport
  x_i : Inport  Port=2  PortDimensions=[3,1]
  u_i : Inport  Port=3  PortDimensions=[3,1]
  Bus Creator : BusCreator  Inputs=2
  Constant : Constant  Value=zeros(6,5)
  First layer : MATLAB Function  TreatAsAtomicUnit=on
  J_hat : Scope
  J_i : Integrator  InitialConditionSource=external
  J_i Initialization : MATLAB Function  TreatAsAtomicUnit=on
  J_i Update : MATLAB Function  TreatAsAtomicUnit=on
  Manual Switch : ManualSwitch  CurrentSetting=0
  Scope : Scope
  Scope1 : Scope
  Second layer : MATLAB Function  TreatAsAtomicUnit=on
  W_hat : Scope
  W_i : Integrator  InitialConditionSource=external
  W_i Initialization : MATLAB Function  TreatAsAtomicUnit=on
  W_i Update : MATLAB Function  TreatAsAtomicUnit=on
  mu : Scope
  w_hat : Outport
  wires:
  e_xi/1 -> W_i Update/1(e_xi), J_i Update/1(e_xi)
  W_i/1 -> W_hat/1, Second layer/1(W_hat), W_i Update/2(W_hat), J_i Update/2(W_hat)
  W_i Update/1(W_dot) -> Scope1/1, W_i/1
  W_i Initialization/1(W_0) -> W_i/2
  J_i Initialization/1(J_0) -> J_i/2
  First layer/1(mu) -> mu/1, Second layer/2(mu), W_i Update/3(mu)
  Second layer/1(w_hat) -> w_hat/1
  J_i/1 -> J_i Update/3(J_hat), J_hat/1, First layer/1(J_hat)
  Bus Creator/1 -> Scope/1, First layer/2(x_bar), J_i Update/4(x_bar)
  x_i/1 -> Bus Creator/1
  u_i/1 -> Bus Creator/2
  J_i Update/1(J_dot) -> Manual Switch/2
  Constant/1 -> Manual Switch/1
  Manual Switch/1 -> J_i/1

== matlab function FO_CTDNN_P_Bia_Para_0_V1/Controller and Plant 1/Smooth Projection ==
  data: u_i input; u_i output
function u_i = fcn(u_i)

tau_i = 0.24;
psi = 0.01;

dimension = 3;

for i = 1 : dimension
   if abs(u_i(i)) <= tau_i
       continue;
   else
       u_i(i) = sign(u_i(i)) * (tau_i + psi*exp((tau_i - abs(u_i(i)))/psi ));
   end 
end



end

== matlab function FO_CTDNN_P_Bia_Para_0_V1/Controller and Plant 1/Local Error Calculate ==
  data: delta_x input; e_xi output; L input
function e_xi = local_error(delta_x, L)

%% Calculate the local formation tracking error from communication

dimension = 3;
serial_num = 1;

L_i = kron(L(serial_num, :) , eye(dimension));

e_xi = L_i * delta_x;







end

== matlab function FO_CTDNN_P_Bia_Para_0_V1/Controller and Plant 2/Local Error Calculate ==
  data: delta_x input; e_xi output; L input
function e_xi = local_error(delta_x, L)

%% Calculate the local formation tracking error from communication

dimension = 3;
serial_num = 2;

L_i = kron(L(serial_num, :) , eye(dimension));

e_xi = L_i * delta_x;







end

== matlab function FO_CTDNN_P_Bia_Para_0_V1/Controller and Plant 2/Multi-layer neural network/First layer ==
  data: J_hat input; mu output; x_bar input
function mu = first_layer(J_hat, x_bar)

%% From input layer to hidden layer
% mu = tanh(J_hat * x_i)

mu = tanh(J_hat' * x_bar);

end

== matlab function FO_CTDNN_P_Bia_Para_0_V1/Controller and Plant 2/Multi-layer neural network/J_i Initialization ==
  data: J_0 output
function J_0 = J_ini()

n_1 = 5;
dimension = 3;

J_0 = rand(2*dimension,n_1);

end

== matlab function FO_CTDNN_P_Bia_Para_0_V1/Controller and Plant 2/Multi-layer neural network/J_i Update ==
  data: e_xi input; J_dot output; W_hat input; J_hat input; x_bar input
function J_dot = J_update(e_xi, W_hat, J_hat, x_bar)


eta_3 = 0.1;
eta_4 = 0.06;
% eta_5 = 0.1;

n_1 = 5;

alpha = tanh(J_hat' * x_bar);

% J_dot = eta_3 * sign(x_bar) * ( e_xi' * W_hat' * (eye(n_1) - diag(alpha.^2)) ) - eta_4 * norm(e_xi) * J_hat - eta_5  * J_hat; 

J_dot = eta_3 * sign(x_bar) * ( e_xi' * W_hat' * (eye(n_1) - diag(alpha.^2)) ) - eta_4 * norm(e_xi) * J_hat; 

% J_dot = eta_3 * sign(x_bar) * ( e_xi' * W_hat' * (eye(n_1) - diag(alpha.^2)) ) - eta_4  * J_hat; 

end

== matlab function FO_CTDNN_P_Bia_Para_0_V1/Controller and Plant 1/controller ==
  data: v_di input; e_xi input; u_i output; w_hat input; x_i input
function u_i  = controller(v_di, e_xi, w_hat, x_i)


%% basic data
Radius_esti=[0.21;0.25;0.33;0.24;0.28;0.29];

serial_num = 1;
dimension = 3; 

R_hat=Radius_esti(serial_num);

theta = x_i(dimension);
k_p = 3;

g_i = [-sin(theta) -sin(pi/3 - theta) sin(pi/3 + theta);
        cos(theta) -cos(pi/3 - theta) -cos(pi/3+ theta);
        1/R_hat 1/R_hat 1/R_hat];

%% First, we apply the smooth projection for uncertainty estimation
% psi = 0.01;
% w_m = 0.10;
% 
% for i = 1 : dimension
%    if abs(w_hat(i)) <= w_m - psi
%        continue;
%    else
%        w_hat(i) = sign(w_hat(i)) * (w_m - psi*exp( (w_m - psi - abs(w_hat(i)))/psi ));
%    end 
% end


u_i = (g_i)^(-1) * (- w_hat + v_di - k_p * e_xi); 




end

== matlab function FO_CTDNN_P_Bia_Para_0_V1/Controller and Plant 2/Multi-layer neural network/Second layer ==
  data: W_hat input; w_hat output; mu input
function w_hat = second_layer(W_hat, mu)

%% From hidden layer to output layer
% w_hat = W_hat * mu(J_hat * x_i)


w_hat = W_hat' * mu; 

end

== matlab function FO_CTDNN_P_Bia_Para_0_V1/Controller and Plant 2/Multi-layer neural network/W_i Initialization ==
  data: W_0 output
function W_0 = W_ini()

n_1 = 5;
dimension = 3;

W_0 = 0.05*zeros(n_1,dimension);
% W_0 =randn(n, n_1);

end

== matlab function FO_CTDNN_P_Bia_Para_0_V1/Controller and Plant 2/Multi-layer neural network/W_i Update ==
  data: e_xi input; W_dot output; W_hat input; mu input
function W_dot = W_update(e_xi, W_hat, mu)


eta_1 = 15;
eta_2 = 0.1;
% eta_3 = 0.05;



% W_dot = eta_1 * mu * e_xi' - eta_2* norm(e_xi) * W_hat - eta_3 * W_hat; 

W_dot = eta_1 * mu * e_xi' - eta_2* norm(e_xi) * W_hat; 

% W_dot = eta_1 * mu * e_xi' - eta_2 * W_hat; 

end

== matlab function FO_CTDNN_P_Bia_Para_0_V1/Controller and Plant 2/Plant ==
  data: x_dot output; E_i output; x_i input; u_i input; t input
function [x_dot, E_i ] = model( x_i, u_i, t)

%% First-order plants for robots

Radius=[0.24;0.23;0.30;0.28;0.25;0.32];
Radius_esti=[0.21;0.25;0.33;0.24;0.28;0.29];

serial_num = 2;
dimension = 3; 

R = Radius(serial_num);
R_hat = Radius_esti(serial_num);

x = x_i(1);
y = x_i(2);
theta = x_i(3);

w_i =  [0.02 * cos(0.5* t+ pi/2) + 0.03 * exp( -abs(x) - 1 ) ; 0.03 * sin(0.2*t) + 0.02*tanh(y); 0.04*sin(0.1*t + theta) + 0.01 *tanh(theta)] ;
%d =  0.4* cos(0.5* t+ pi/2);


g_i = [-sin(theta) -sin(pi/3 - theta) sin(pi/3 + theta);
        cos(theta) -cos(pi/3 - theta) -cos(pi/3+ theta);
        1/R 1/R 1/R];
    
g_i_hat = [-sin(theta) -sin(pi/3 - theta) sin(pi/3 + theta);
        cos(theta) -cos(pi/3 - theta) -cos(pi/3+ theta);
        1/R_hat 1/R_hat 1/R_hat];
    
x_dot = g_i * u_i + w_i;


E_i = w_i + (g_i - g_i_hat) * u_i;




end

== matlab function FO_CTDNN_P_Bia_Para_0_V1/Self Error Calculation 2/error_calculation ==
  data: v_di output; ref input; delta_x2 output; x_i input
function [v_di, delta_x2] = error_cal(ref, x_i)

%% Basic parameters

dimension = 3;
num_agent = 6;
serial_num = 2;

x_d = ref(1+dimension*0:dimension*num_agent);
v_d = ref(1+dimension*num_agent:2*dimension*num_agent);

x_di = x_d( (serial_num - 1)*dimension+1 : serial_num*dimension );
v_di = v_d( (serial_num - 1)*dimension+1 : serial_num*dimension );



delta_x2 = x_i - x_di;


end

== matlab function FO_CTDNN_P_Bia_Para_0_V1/Controller and Plant 2/Smooth Projection ==
  data: u_i input; u_i output
function u_i = fcn(u_i)

tau_i = 0.24;
psi = 0.01;

dimension = 3;

for i = 1 : dimension
   if abs(u_i(i)) <= tau_i
       continue;
   else
       u_i(i) = sign(u_i(i)) * (tau_i + psi*exp((tau_i - abs(u_i(i)))/psi ));
   end 
end



end

== matlab function FO_CTDNN_P_Bia_Para_0_V1/Controller and Plant 2/controller ==
  data: v_di input; e_xi input; u_i output; w_hat input; x_i input
function u_i  = controller(v_di, e_xi, w_hat, x_i)


%% basic data
Radius_esti=[0.21;0.25;0.33;0.24;0.28;0.29];

serial_num = 2;
dimension = 3; 

R_hat=Radius_esti(serial_num);

theta = x_i(dimension);
k_p = 3;

g_i = [-sin(theta) -sin(pi/3 - theta) sin(pi/3 + theta);
        cos(theta) -cos(pi/3 - theta) -cos(pi/3+ theta);
        1/R_hat 1/R_hat 1/R_hat];

%% First, we apply the smooth projection for uncertainty estimation
% psi = 0.01;
% w_m = 0.10;
% 
% for i = 1 : dimension
%    if abs(w_hat(i)) <= w_m - psi
%        continue;
%    else
%        w_hat(i) = sign(w_hat(i)) * (w_m - psi*exp( (w_m - psi - abs(w_hat(i)))/psi ));
%    end 
% end


u_i = (g_i)^(-1) * (- w_hat + v_di - k_p * e_xi); 




end

== matlab function FO_CTDNN_P_Bia_Para_0_V1/Controller and Plant 3/Local Error Calculate ==
  data: delta_x input; e_xi output; L input
function e_xi = local_error(delta_x, L)

%% Calculate the local formation tracking error from communication

dimension = 3;
serial_num = 3;

L_i = kron(L(serial_num, :) , eye(dimension));

e_xi = L_i * delta_x;







end

== matlab function FO_CTDNN_P_Bia_Para_0_V1/Controller and Plant 3/Multi-layer neural network/First layer ==
  data: J_hat input; mu output; x_bar input
function mu = first_layer(J_hat, x_bar)

%% From input layer to hidden layer
% mu = tanh(J_hat * x_i)

mu = tanh(J_hat' * x_bar);

end

== matlab function FO_CTDNN_P_Bia_Para_0_V1/Controller and Plant 3/Multi-layer neural network/J_i Initialization ==
  data: J_0 output
function J_0 = J_ini()

n_1 = 5;
dimension = 3;

J_0 = rand(2*dimension,n_1);

end

== matlab function FO_CTDNN_P_Bia_Para_0_V1/Controller and Plant 3/Multi-layer neural network/J_i Update ==
  data: e_xi input; J_dot output; W_hat input; J_hat input; x_bar input
function J_dot = J_update(e_xi, W_hat, J_hat, x_bar)


eta_3 = 0.1;
eta_4 = 0.06;
% eta_5 = 0.1;

n_1 = 5;

alpha = tanh(J_hat' * x_bar);

% J_dot = eta_3 * sign(x_bar) * ( e_xi' * W_hat' * (eye(n_1) - diag(alpha.^2)) ) - eta_4 * norm(e_xi) * J_hat - eta_5  * J_hat; 

J_dot = eta_3 * sign(x_bar) * ( e_xi' * W_hat' * (eye(n_1) - diag(alpha.^2)) ) - eta_4 * norm(e_xi) * J_hat; 

% J_dot = eta_3 * sign(x_bar) * ( e_xi' * W_hat' * (eye(n_1) - diag(alpha.^2)) ) - eta_4  * J_hat; 

end

== matlab function FO_CTDNN_P_Bia_Para_0_V1/Controller and Plant 3/Multi-layer neural network/Second layer ==
  data: W_hat input; w_hat output; mu input
function w_hat = second_layer(W_hat, mu)

%% From hidden layer to output layer
% w_hat = W_hat * mu(J_hat * x_i)


w_hat = W_hat' * mu; 

end

== matlab function FO_CTDNN_P_Bia_Para_0_V1/Controller and Plant 1/Plant ==
  data: x_dot output; E_i output; x_i input; u_i input; t input
function [x_dot, E_i ] = model( x_i, u_i, t)

%% First-order plants for robots

Radius=[0.24;0.23;0.30;0.28;0.25;0.32];
Radius_esti=[0.21;0.25;0.33;0.24;0.28;0.29];

serial_num = 1;
dimension = 3; 

R = Radius(serial_num);
R_hat = Radius_esti(serial_num);

x = x_i(1);
y = x_i(2);
theta = x_i(3);

w_i =  [0.02 * cos(0.5* t+ pi/2) + 0.03 * exp( -abs(x) - 1 ) ; 0.03 * sin(0.2*t) + 0.02*tanh(y); 0.04*sin(0.1*t + theta) + 0.01 *tanh(theta)] ;
%d =  0.4* cos(0.5* t+ pi/2);


g_i = [-sin(theta) -sin(pi/3 - theta) sin(pi/3 + theta);
        cos(theta) -cos(pi/3 - theta) -cos(pi/3+ theta);
        1/R 1/R 1/R];
    
g_i_hat = [-sin(theta) -sin(pi/3 - theta) sin(pi/3 + theta);
        cos(theta) -cos(pi/3 - theta) -cos(pi/3+ theta);
        1/R_hat 1/R_hat 1/R_hat];
    
x_dot = g_i * u_i + w_i;


E_i = w_i + (g_i - g_i_hat) * u_i;




end

== matlab function FO_CTDNN_P_Bia_Para_0_V1/Controller and Plant 3/Multi-layer neural network/W_i Initialization ==
  data: W_0 output
function W_0 = W_ini()

n_1 = 5;
dimension = 3;

W_0 = 0.05*zeros(n_1,dimension);
% W_0 =randn(n, n_1);

end

== matlab function FO_CTDNN_P_Bia_Para_0_V1/Controller and Plant 3/Multi-layer neural network/W_i Update ==
  data: e_xi input; W_dot output; W_hat input; mu input
function W_dot = W_update(e_xi, W_hat, mu)


eta_1 = 15;
eta_2 = 0.1;
% eta_3 = 0.05;



% W_dot = eta_1 * mu * e_xi' - eta_2* norm(e_xi) * W_hat - eta_3 * W_hat; 

W_dot = eta_1 * mu * e_xi' - eta_2* norm(e_xi) * W_hat; 

% W_dot = eta_1 * mu * e_xi' - eta_2 * W_hat; 

end

== matlab function FO_CTDNN_P_Bia_Para_0_V1/Self Error Calculation 3/error_calculation ==
  data: v_di output; ref input; delta_x3 output; x_i input
function [v_di, delta_x3] = error_cal(ref, x_i)

%% Basic parameters

dimension = 3;
num_agent = 6;
serial_num = 3;

x_d = ref(1+dimension*0:dimension*num_agent);
v_d = ref(1+dimension*num_agent:2*dimension*num_agent);

x_di = x_d( (serial_num - 1)*dimension+1 : serial_num*dimension );
v_di = v_d( (serial_num - 1)*dimension+1 : serial_num*dimension );



delta_x3 = x_i - x_di;


end

== matlab function FO_CTDNN_P_Bia_Para_0_V1/Controller and Plant 3/Plant ==
  data: x_dot output; E_i output; x_i input; u_i input; t input
function [x_dot, E_i ] = model( x_i, u_i, t)

%% First-order plants for robots

Radius=[0.24;0.23;0.30;0.28;0.25;0.32];
Radius_esti=[0.21;0.25;0.33;0.24;0.28;0.29];

serial_num = 3;
dimension = 3; 

R = Radius(serial_num);
R_hat = Radius_esti(serial_num);

x = x_i(1);
y = x_i(2);
theta = x_i(3);

w_i =  [0.02 * cos(0.5* t+ pi/2) + 0.03 * exp( -abs(x) - 1 ) ; 0.03 * sin(0.2*t) + 0.02*tanh(y); 0.04*sin(0.1*t + theta) + 0.01 *tanh(theta)] ;
%d =  0.4* cos(0.5* t+ pi/2);


g_i = [-sin(theta) -sin(pi/3 - theta) sin(pi/3 + theta);
        cos(theta) -cos(pi/3 - theta) -cos(pi/3+ theta);
        1/R 1/R 1/R];
    
g_i_hat = [-sin(theta) -sin(pi/3 - theta) sin(pi/3 + theta);
        cos(theta) -cos(pi/3 - theta) -cos(pi/3+ theta);
        1/R_hat 1/R_hat 1/R_hat];
    
x_dot = g_i * u_i + w_i;


E_i = w_i + (g_i - g_i_hat) * u_i;




end

== matlab function FO_CTDNN_P_Bia_Para_0_V1/Controller and Plant 3/Smooth Projection ==
  data: u_i input; u_i output
function u_i = fcn(u_i)

tau_i = 0.24;
psi = 0.01;

dimension = 3;

for i = 1 : dimension
   if abs(u_i(i)) <= tau_i
       continue;
   else
       u_i(i) = sign(u_i(i)) * (tau_i + psi*exp((tau_i - abs(u_i(i)))/psi ));
   end 
end



end

== matlab function FO_CTDNN_P_Bia_Para_0_V1/Controller and Plant 3/controller ==
  data: v_di input; e_xi input; u_i output; w_hat input; x_i input
function u_i  = controller(v_di, e_xi, w_hat, x_i)


%% basic data
Radius_esti=[0.21;0.25;0.33;0.24;0.28;0.29];

serial_num = 3;
dimension = 3; 

R_hat=Radius_esti(serial_num);

theta = x_i(dimension);
k_p = 3;

g_i = [-sin(theta) -sin(pi/3 - theta) sin(pi/3 + theta);
        cos(theta) -cos(pi/3 - theta) -cos(pi/3+ theta);
        1/R_hat 1/R_hat 1/R_hat];

%% First, we apply the smooth projection for uncertainty estimation
% psi = 0.01;
% w_m = 0.10;
% 
% for i = 1 : dimension
%    if abs(w_hat(i)) <= w_m - psi
%        continue;
%    else
%        w_hat(i) = sign(w_hat(i)) * (w_m - psi*exp( (w_m - psi - abs(w_hat(i)))/psi ));
%    end 
% end

u_i = (g_i)^(-1) * (- w_hat + v_di - k_p * e_xi); 




end

== matlab function FO_CTDNN_P_Bia_Para_0_V1/Controller and Plant 4/Local Error Calculate ==
  data: delta_x input; e_xi output; L input
function e_xi = local_error(delta_x, L)

%% Calculate the local formation tracking error from communication

dimension = 3;
serial_num = 4;

L_i = kron(L(serial_num, :) , eye(dimension));

e_xi = L_i * delta_x;







end

== matlab function FO_CTDNN_P_Bia_Para_0_V1/Controller and Plant 4/Multi-layer neural network/First layer ==
  data: J_hat input; mu output; x_bar input
function mu = first_layer(J_hat, x_bar)

%% From input layer to hidden layer
% mu = tanh(J_hat * x_i)

mu = tanh(J_hat' * x_bar);

end

== matlab function FO_CTDNN_P_Bia_Para_0_V1/Controller and Plant 4/Multi-layer neural network/J_i Initialization ==
  data: J_0 output
function J_0 = J_ini()

n_1 = 5;
dimension = 3;

J_0 = rand(2*dimension,n_1);

end

== matlab function FO_CTDNN_P_Bia_Para_0_V1/Controller and Plant 4/Multi-layer neural network/J_i Update ==
  data: e_xi input; J_dot output; W_hat input; J_hat input; x_bar input
function J_dot = J_update(e_xi, W_hat, J_hat, x_bar)


eta_3 = 0.1;
eta_4 = 0.06;
% eta_5 = 0.1;

n_1 = 5;

alpha = tanh(J_hat' * x_bar);

% J_dot = eta_3 * sign(x_bar) * ( e_xi' * W_hat' * (eye(n_1) - diag(alpha.^2)) ) - eta_4 * norm(e_xi) * J_hat - eta_5  * J_hat; 

J_dot = eta_3 * sign(x_bar) * ( e_xi' * W_hat' * (eye(n_1) - diag(alpha.^2)) ) - eta_4 * norm(e_xi) * J_hat; 

% J_dot = eta_3 * sign(x_bar) * ( e_xi' * W_hat' * (eye(n_1) - diag(alpha.^2)) ) - eta_4  * J_hat; 

end

== matlab function FO_CTDNN_P_Bia_Para_0_V1/Controller and Plant 4/Multi-layer neural network/Second layer ==
  data: W_hat input; w_hat output; mu input
function w_hat = second_layer(W_hat, mu)

%% From hidden layer to output layer
% w_hat = W_hat * mu(J_hat * x_i)


w_hat = W_hat' * mu; 

end

== matlab function FO_CTDNN_P_Bia_Para_0_V1/Controller and Plant 4/Multi-layer neural network/W_i Initialization ==
  data: W_0 output
function W_0 = W_ini()

n_1 = 5;
dimension = 3;

W_0 = 0.05*zeros(n_1,dimension);
% W_0 =randn(n, n_1);

end

== matlab function FO_CTDNN_P_Bia_Para_0_V1/Self Error Calculation 4/error_calculation ==
  data: v_di output; ref input; delta_x4 output; x_i input
function [v_di, delta_x4] = error_cal(ref, x_i)

%% Basic parameters

dimension = 3;
num_agent = 6;
serial_num = 4;

x_d = ref(1+dimension*0:dimension*num_agent);
v_d = ref(1+dimension*num_agent:2*dimension*num_agent);

x_di = x_d( (serial_num - 1)*dimension+1 : serial_num*dimension );
v_di = v_d( (serial_num - 1)*dimension+1 : serial_num*dimension );



delta_x4 = x_i - x_di;


end

== matlab function FO_CTDNN_P_Bia_Para_0_V1/Self Error Calculation 1/error_calculation ==
  data: v_di output; ref input; delta_x1 output; x_i input
function [v_di, delta_x1] = error_cal(ref, x_i)

%% Basic parameters

dimension = 3;
num_agent = 6;
serial_num = 1;

x_d = ref(1+dimension*0:dimension*num_agent);
v_d = ref(1+dimension*num_agent:2*dimension*num_agent);

x_di = x_d( (serial_num - 1)*dimension+1 : serial_num*dimension );
v_di = v_d( (serial_num - 1)*dimension+1 : serial_num*dimension );



delta_x1 = x_i - x_di;


end

== matlab function FO_CTDNN_P_Bia_Para_0_V1/Controller and Plant 4/Multi-layer neural network/W_i Update ==
  data: e_xi input; W_dot output; W_hat input; mu input
function W_dot = W_update(e_xi, W_hat, mu)


eta_1 = 15;
eta_2 = 0.1;
% eta_3 = 0.05;



% W_dot = eta_1 * mu * e_xi' - eta_2* norm(e_xi) * W_hat - eta_3 * W_hat; 

W_dot = eta_1 * mu * e_xi' - eta_2* norm(e_xi) * W_hat; 

% W_dot = eta_1 * mu * e_xi' - eta_2 * W_hat; 

end

== matlab function FO_CTDNN_P_Bia_Para_0_V1/Controller and Plant 4/Plant ==
  data: x_dot output; E_i output; x_i input; u_i input; t input
function [x_dot, E_i ] = model( x_i, u_i, t)

%% First-order plants for robots

Radius=[0.24;0.23;0.30;0.28;0.25;0.32];
Radius_esti=[0.21;0.25;0.33;0.24;0.28;0.29];

serial_num = 4;
dimension = 3; 

R = Radius(serial_num);
R_hat = Radius_esti(serial_num);

x = x_i(1);
y = x_i(2);
theta = x_i(3);

w_i =  [0.02 * cos(0.5* t+ pi/2) + 0.03 * exp( -abs(x) - 1 ) ; 0.03 * sin(0.2*t) + 0.02*tanh(y); 0.04*sin(0.1*t + theta) + 0.01 *tanh(theta)] ;
%d =  0.4* cos(0.5* t+ pi/2);


g_i = [-sin(theta) -sin(pi/3 - theta) sin(pi/3 + theta);
        cos(theta) -cos(pi/3 - theta) -cos(pi/3+ theta);
        1/R 1/R 1/R];
    
g_i_hat = [-sin(theta) -sin(pi/3 - theta) sin(pi/3 + theta);
        cos(theta) -cos(pi/3 - theta) -cos(pi/3+ theta);
        1/R_hat 1/R_hat 1/R_hat];
    
x_dot = g_i * u_i + w_i;


E_i = w_i + (g_i - g_i_hat) * u_i;




end

== matlab function FO_CTDNN_P_Bia_Para_0_V1/Controller and Plant 4/Smooth Projection ==
  data: u_i input; u_i output
function u_i = fcn(u_i)

tau_i = 0.24;
psi = 0.01;

dimension = 3;

for i = 1 : dimension
   if abs(u_i(i)) <= tau_i
       continue;
   else
       u_i(i) = sign(u_i(i)) * (tau_i + psi*exp((tau_i - abs(u_i(i)))/psi ));
   end 
end



end

== matlab function FO_CTDNN_P_Bia_Para_0_V1/Controller and Plant 4/controller ==
  data: v_di input; e_xi input; u_i output; w_hat input; x_i input
function u_i  = controller(v_di, e_xi, w_hat, x_i)


%% basic data
Radius_esti=[0.21;0.25;0.33;0.24;0.28;0.29];

serial_num = 4;
dimension = 3; 

R_hat=Radius_esti(serial_num);

theta = x_i(dimension);
k_p = 3;

g_i = [-sin(theta) -sin(pi/3 - theta) sin(pi/3 + theta);
        cos(theta) -cos(pi/3 - theta) -cos(pi/3+ theta);
        1/R_hat 1/R_hat 1/R_hat];

%% First, we apply the smooth projection for uncertainty estimation
% psi = 0.01;
% w_m = 0.10;
% 
% for i = 1 : dimension
%    if abs(w_hat(i)) <= w_m - psi
%        continue;
%    else
%        w_hat(i) = sign(w_hat(i)) * (w_m - psi*exp( (w_m - psi - abs(w_hat(i)))/psi ));
%    end 
% end

u_i = (g_i)^(-1) * (- w_hat + v_di - k_p * e_xi); 




end

== matlab function FO_CTDNN_P_Bia_Para_0_V1/Controller and Plant 5/Local Error Calculate ==
  data: delta_x input; e_xi output; L input
function e_xi = local_error(delta_x, L)

%% Calculate the local formation tracking error from communication

dimension = 3;
serial_num = 5;

L_i = kron(L(serial_num, :) , eye(dimension));

e_xi = L_i * delta_x;







end

== matlab function FO_CTDNN_P_Bia_Para_0_V1/Controller and Plant 5/Multi-layer neural network/First layer ==
  data: J_hat input; mu output; x_bar input
function mu = first_layer(J_hat, x_bar)

%% From input layer to hidden layer
% mu = tanh(J_hat * x_i)

mu = tanh(J_hat' * x_bar);

end

== matlab function FO_CTDNN_P_Bia_Para_0_V1/Controller and Plant 5/Multi-layer neural network/J_i Initialization ==
  data: J_0 output
function J_0 = J_ini()

n_1 = 5;
dimension = 3;

J_0 = rand(2*dimension,n_1);

end

== matlab function FO_CTDNN_P_Bia_Para_0_V1/Controller and Plant 5/Multi-layer neural network/J_i Update ==
  data: e_xi input; J_dot output; W_hat input; J_hat input; x_bar input
function J_dot = J_update(e_xi, W_hat, J_hat, x_bar)


eta_3 = 0.1;
eta_4 = 0.06;
% eta_5 = 0.1;

n_1 = 5;

alpha = tanh(J_hat' * x_bar);

% J_dot = eta_3 * sign(x_bar) * ( e_xi' * W_hat' * (eye(n_1) - diag(alpha.^2)) ) - eta_4 * norm(e_xi) * J_hat - eta_5  * J_hat; 

J_dot = eta_3 * sign(x_bar) * ( e_xi' * W_hat' * (eye(n_1) - diag(alpha.^2)) ) - eta_4 * norm(e_xi) * J_hat; 

% J_dot = eta_3 * sign(x_bar) * ( e_xi' * W_hat' * (eye(n_1) - diag(alpha.^2)) ) - eta_4  * J_hat; 

end

== matlab function FO_CTDNN_P_Bia_Para_0_V1/Controller and Plant 5/Multi-layer neural network/Second layer ==
  data: W_hat input; w_hat output; mu input
function w_hat = second_layer(W_hat, mu)

%% From hidden layer to output layer
% w_hat = W_hat * mu(J_hat * x_i)


w_hat = W_hat' * mu; 

end

== matlab function FO_CTDNN_P_Bia_Para_0_V1/Self Error Calculation 5/error_calculation ==
  data: v_di output; ref input; delta_x5 output; x_i input
function [v_di, delta_x5] = error_cal(ref, x_i)

%% Basic parameters

dimension = 3;
num_agent = 6;
serial_num = 5;

x_d = ref(1+dimension*0:dimension*num_agent);
v_d = ref(1+dimension*num_agent:2*dimension*num_agent);

x_di = x_d( (serial_num - 1)*dimension+1 : serial_num*dimension );
v_di = v_d( (serial_num - 1)*dimension+1 : serial_num*dimension );



delta_x5 = x_i - x_di;


end
